simulink library "tether001_cl"  (R2020a)
settings: Solver=VariableStepAuto  StartTime=0.0  StopTime=10.0  RelTol=1e-3
undefined symbols (not defined in the file or in its folder): env, initNodePos, minLinkDeviation, minLinkLength, minSoftLength, numNodes, thr
libraries: powerlib_meascontrol x1, nodePosToLinkPos_ul x1
settings Model: Creator=mr-jo  LastModifiedBy=John Jr

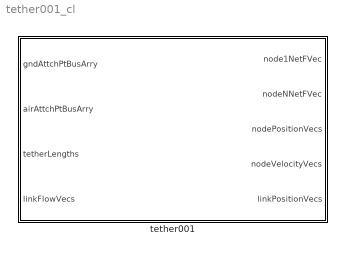
== system tether001_cl ==
  tether001 : Subsystem  mask{thr=thr.tether1, fluidDensity=env.water.density.Value, gravity=env.gravAccel.Value}
      mask prompts: thr "Tether001 Object"; fluidDensity "Fluid Density"; gravity "Gravitational Aceleration"

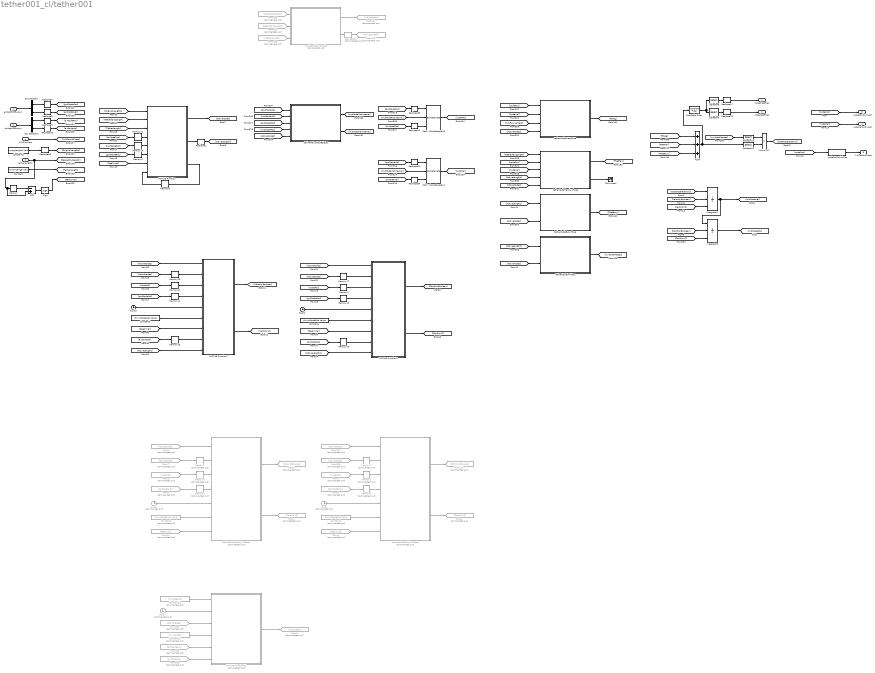
== system tether001_cl/tether001 ==
  gndAttchPtBusArry : Inport  OutDataTypeStr=Bus: thrAttachPtKinematicsBus
  airAttchPtBusArry : Inport  Port=2  OutDataTypeStr=Bus: thrAttachPtKinematicsBus
  tetherLengths : Inport  Port=3
  linkFlowVecs : Inport  Port=4
  Add : Sum  Inputs=-+
  Add4 : Sum  Inputs=3
  Bus Selector : BusSelector  OutputSignals=posVec,velVec
  Bus Selector1 : BusSelector  OutputSignals=posVec,velVec
  Clock : Clock  Commented=on
  Clock1 : Clock  Commented=on
  Clock2 : Clock
  Clock3 : Clock
  Clock7 : Clock  Commented=on
  Constant : Constant  Value=thr.maxLength.Value
  Constant1 : Constant  Commented=on  Value=thr.initNodePos.Value
  Constant15 : Constant  Commented=on  Value=[initNodePos]
  Constant19 : Constant  Commented=on  Value=[numNodes]
  Constant2 : Constant  Commented=on  Value=thr.initNodeVel.Value
  Constant3 : Constant  Value=thr.orgLengths.Value
  Constant4 : Constant  Value=thr.initNodePos.Value
  Constant5 : Constant  Value=thr.initNodeVel.Value
  First-Order Filter : powerlib_meascontrol/Filters/First-Order Filter  FilterType=Lowpass  Tc=10e-2  Ts=0  Initialize=on  Vac_Init=[0, 0, 60]  Vdc_Init=0  PlotResponse=off  FreqRange="[0,  200,  1]"
  From1 : From  Commented=on  GotoTag=nodePos
  From10 : From  Commented=on  GotoTag=ReelInVel
  From161 : From  Commented=on  GotoTag=gndNodePos
  From162 : From  Commented=on  GotoTag=airNodePos
  From2 : From  Commented=on  GotoTag=gndNodePos
  From{4,7,267..268,361} (5 alike) : From  Commented=on  GotoTag=ActiveNodes
  From310 : From  Commented=on  GotoTag=OriginalLengths
  From311 : From  Commented=on  GotoTag=ReeledOutLength
  From320 : From  Commented=on  GotoTag=TetherLength
  From5 : From  Commented=on  GotoTag=ReelInVel
  From8 : From  Commented=on  GotoTag=nodeVel
  From9 : From  Commented=on  GotoTag=gndNodeVel
  Goto110 : Goto  Commented=on  GotoTag=PositionBoolean
  Goto152 : Goto  Commented=on  GotoTag=ActiveLengths
  Goto161 : Goto  Commented=on  GotoTag=ActiveNodes
  Goto2 : Goto  Commented=on  GotoTag=PositionIC
  Goto3 : Goto  Commented=on  GotoTag=VelocityBoolean
  Goto4 : Goto  Commented=on  GotoTag=VelocityIC
  Goto5 : Goto  Commented=on  GotoTag=PosIC_Start
  Integrator1 : Integrator  ExternalReset=rising  InitialConditionSource=external
  Integrator8 : Integrator  ExternalReset=rising  InitialConditionSource=external
  MATLAB Function : MATLAB Function  TreatAsAtomicUnit=on  mask{minLinkLength=minLinkLength, minLinkDeviation=minLinkDeviation}
      mask prompts: minLinkLength "Minimum Link Length"; minLinkDeviation "Minimum Devation to Remove Node"
  MATLAB Function1 : MATLAB Function  TreatAsAtomicUnit=on
  MATLAB Function2 : MATLAB Function  TreatAsAtomicUnit=on
  MATLAB Function61 : MATLAB Function  Commented=on  TreatAsAtomicUnit=on
  Matrix Concatenate14 : Concatenate  NumInputs=3  Mode=Multidimensional array  ConcatenateDimension=2
  Matrix Concatenate15 : Concatenate  NumInputs=3  Mode=Multidimensional array  ConcatenateDimension=2
  Memory{,6,8..18} (13 alike) : Memory
  Memory{1..5,7} (6 alike) : Memory  Commented=on
  Multiply11 : Product
  Reshape1 : Reshape  OutputDimensionality=Row vector (2-D)
  Reshape{7..10,17..18,33..34,41..42} (10 alike) : Reshape  OutputDimensionality=Column vector (2-D)
  Reshape36 : Reshape  OutputDimensionality=Row vector (2-D)
  Reshape39 : Reshape  Commented=on  OutputDimensionality=Row vector (2-D)
  Selector18 : Selector  NumberOfDimensions=2  InputPortWidth=3  IndexOptions=Select all,Index vector (dialog)  Indices=[1 3],2:thr.numNodes.Value-1  OutputSizes=1,1
  Selector19 : Selector  NumberOfDimensions=2  InputPortWidth=3  IndexOptions=Select all,Index vector (dialog)  Indices=[1 3],2:thr.numNodes.Value-1  OutputSizes=1,1
  Selector8 : Selector  NumberOfDimensions=2  InputPortWidth=3  IndexOptions=Select all,Index vector (dialog)  Indices=[1 3],1  OutputSizes=1,1
  Selector9 : Selector  NumberOfDimensions=2  InputPortWidth=3  IndexOptions=Select all,Starting index (dialog)  Indices=[1 3],thr.numNodes.Value  OutputSizes=1,1
  Sign : Signum
  Terminator : Terminator
  defineActiveNodeStates : MATLAB Function  TreatAsAtomicUnit=on
  nodePosToLinkPos : nodePosToLinkPos_ul/nodePosToLinkPos  SystemSampleTime=-1  Latency=0  AutoFrameSizeCalculation=off
  numberOfActiveNodes : MATLAB Function  Commented=on  TreatAsAtomicUnit=on
  tetherNodeBuoyForce : MATLAB Function  TreatAsAtomicUnit=on  mask{fluidDensity=fluidDensity, numNodes=thr.numNodes.Value, thrDiam=thr.diameter.Value, tetherDensity=thr.density.Value, gravity=gravity}
      mask prompts: fluidDensity "Fluid Density"; numNodes "Number of Nodes"; thrDiam "Tether Diameter"; tetherDensity "Tether Density"; gravity "Gravitational Acceleration"
  tetherNodeDragForce : MATLAB Function  TreatAsAtomicUnit=on  mask{flowDensity=fluidDensity, numNodes=thr.numNodes.Value, dragCoeff=thr.dragCoeff.Value, thrDiam=thr.diameter.Value}
      mask prompts: flowDensity "Fluid Density"; numNodes "Number of nodes"; dragCoeff "Drag Coefficient of Tether"; thrDiam "Tether Diameter"
  tetherNodeInvMass : MATLAB Function  TreatAsAtomicUnit=on  mask{numNodes=thr.numNodes.Value, thrDiam=thr.diameter.Value, tetherDensity=thr.density.Value}
      mask prompts: numNodes "Number of nodes"; thrDiam "Tether Diameter"; tetherDensity "Tether Density"
  tetherNodePositionICReset : MATLAB Function  Commented=on  TreatAsAtomicUnit=on
  tetherNodeTensionForce : MATLAB Function  TreatAsAtomicUnit=on  mask{numNodes=thr.numNodes.Value, thrDiam=thr.diameter.Value, youngsMod=thr.youngsMod.Value, dampingRatio=thr.dampingRatio.Value, mass=thr.vehicleMass.Value, minSoftLength=minSoftLength}
      mask prompts: numNodes "Number of Nodes"; thrDiam "Tether Diameter"; youngsMod "Youngs Modulus of Tether"; dampingRatio "Total Tether Damping Ratio"; mass "Vehicle Mass for Damping"; minSoftLength "Min Link Length for Spring Softening"
  tetherNodeVelocityICReset : MATLAB Function  Commented=on  TreatAsAtomicUnit=on
  node1NetFVec : Outport  VectorParamsAs1DForOutWhenUnconnected=off
  nodeNNetFVec : Outport  Port=2  VectorParamsAs1DForOutWhenUnconnected=off
  nodePositionVecs : Outport  Port=3  VectorParamsAs1DForOutWhenUnconnected=off
  nodeVelocityVecs : Outport  Port=4  VectorParamsAs1DForOutWhenUnconnected=off
  linkPositionVecs : Outport  Port=5  VectorParamsAs1DForOutWhenUnconnected=off
  wires:
  [nodePos] -> nodePosToLinkPos/1
  nodePosToLinkPos/1 -> linkPositionVecs/1  "linkPositions"
  [nodeVel] -> nodeVelocityVecs/1
  [nodePos] -> nodePositionVecs/1
  Constant3/1 -> Reshape36/1
  Sign/1 -> [ReelInVel]
  Add/1 -> Sign/1
  Memory/1 -> Add/1
  Bus Selector/1 -> Reshape7/1  "<posVec>"
  Reshape8/1 -> [gndNodeVel]
  Bus Selector1/1 -> Reshape9/1  "<posVec>"
  Bus Selector/2 -> Reshape8/1  "<velVec>"
  airAttchPtBusArry/1 -> Bus Selector1/1
  Reshape9/1 -> [airNodePos]
  Reshape10/1 -> [airNodeVel]
  Reshape7/1 -> [gndNodePos]
  gndAttchPtBusArry/1 -> Bus Selector/1
  Bus Selector1/2 -> Reshape10/1  "<velVec>"
  Constant1/1 -> tetherNodePositionICReset/6(GivenIC)
  MATLAB Function61/1(PosIC_Start) -> Goto5/1
  Constant15/1 -> MATLAB Function61/1(initNodePos)
  From161/1 -> MATLAB Function61/5(gndNodePos)
  Clock7/1 -> MATLAB Function61/2(time)
  From162/1 -> MATLAB Function61/6(airNodePos)
  Constant19/1 -> MATLAB Function61/4(OriginalNodes)
  From361/1 -> MATLAB Function61/3(ActiveNodes)
  Memory1/1 -> tetherNodePositionICReset/3(nodePositions)
  From1/1 -> Memory1/1
  [ActiveNodes] -> tetherNodeInvMass/2(ActiveNodes)
  [ActiveLengths] -> tetherNodeBuoyForce/1(ActiveLengths)
  [VelocityBoolean] -> Integrator1/2
  [VelocityIC] -> Integrator1/3
  tetherNodeVelocityICReset/2(VelocityIC) -> Goto4/1
  tetherNodeVelocityICReset/1(Bool) -> Goto3/1
  From10/1 -> tetherNodeVelocityICReset/7(ReelInVel)
  Constant2/1 -> tetherNodeVelocityICReset/6(GivenIC)
  Clock1/1 -> tetherNodeVelocityICReset/5(time)
  Memory5/1 -> tetherNodeVelocityICReset/4(gndNodeVel)
  From9/1 -> Memory5/1
  Memory4/1 -> tetherNodeVelocityICReset/3(nodeVelocities)
  From8/1 -> Memory4/1
  Memory2/1 -> tetherNodeVelocityICReset/2(PrevStepNumNodes)
  From7/1 -> Memory2/1
  From4/1 -> tetherNodeVelocityICReset/1(CurStepNumNodes)
  [PositionBoolean] -> Integrator8/2
  Selector9/1 -> Reshape18/1
  Selector8/1 -> Reshape17/1
  From5/1 -> tetherNodePositionICReset/7(ReelInVel)
  Memory3/1 -> tetherNodePositionICReset/4(gndNodePos)
  [PositionIC] -> Integrator8/3
  Clock/1 -> tetherNodePositionICReset/5(time)
  tetherNodePositionICReset/2(PositionIC) -> Goto2/1
  From2/1 -> Memory3/1
  [NodeAccelerations] -> Integrator1/1
  [FNetBuoy] -> Add4/3  "FbuoyT"
  Multiply11/1 -> [NodeAccelerations]
  [FDrag] -> Add4/1  "FdragT"
  Selector19/1 -> Multiply11/1
  [invNodeMasses] -> Selector19/1
  Memory7/1 -> tetherNodePositionICReset/2(PrevStepNumNodes)
  From268/1 -> Memory7/1
  tetherNodePositionICReset/1(Bool) -> Goto110/1
  From267/1 -> tetherNodePositionICReset/1(CurStepNumNodes)
  defineActiveNodeStates/1(midNodePosInternal) -> [midNodePosInternal]
  Constant/1 -> [TetherLength]
  linkFlowVecs/1 -> [linkFlowVelVecs]
  Reshape36/1 -> [OriginalLengths]
  tetherLengths/1 -> [ReeledOutLength], Memory/1, Add/2
  From310/1 -> numberOfActiveNodes/1(OriginalLengths)
  [linkFlowVelVecs] -> tetherNodeDragForce/3(flowVel)
  [midNodeVel] -> defineActiveNodeStates/2(midNodeVel)
  [nodePos] -> tetherNodeTensionForce/2(nodePos)
  defineActiveNodeStates/2(midNodeVelInternal) -> [midNodeVelInternal]
  [ReeledOutLength] -> tetherNodeTensionForce/1(ReeledOutLength)
  [ActiveNodes] -> tetherNodeDragForce/4(NumberNodesActive)
  From320/1 -> numberOfActiveNodes/3(TetherLength)
  [nodeVel] -> tetherNodeDragForce/2(nodeVelocities)
  Reshape34/1 -> Matrix Concatenate14/3
  [gndNodePos] -> defineActiveNodeStates/3(gndNodePos)
  [midNodeVelInternal] -> Matrix Concatenate14/2
  [ActiveNodes] -> defineActiveNodeStates/5(ActiveNodes)
  [midNodePos] -> defineActiveNodeStates/4(midNodePos)
  numberOfActiveNodes/1(ActiveNodes) -> Goto161/1
  [gndNodeVel] -> defineActiveNodeStates/1(gndNodeVel)
  [ActiveLengths] -> tetherNodeTensionForce/4(ActiveLengths)
  Matrix Concatenate15/1 -> [nodePos]
  tetherNodeTensionForce/1(nodeForceVecs) -> [FNetTen]
  Matrix Concatenate14/1 -> [nodeVel]
  [nodeVel] -> tetherNodeTensionForce/3(nodeVel)
  [airNodeVel] -> Reshape34/1
  Reshape33/1 -> Matrix Concatenate15/1
  Reshape41/1 -> Matrix Concatenate15/3
  Reshape39/1 -> Goto152/1
  [ActiveNodes] -> tetherNodeBuoyForce/2(NumberNodesActive)
  Reshape42/1 -> Matrix Concatenate14/1
  From311/1 -> numberOfActiveNodes/2(ReeledOutLength)
  tetherNodeBuoyForce/1(nodeForceVecs) -> [FNetBuoy]
  [ActiveLengths] -> tetherNodeInvMass/1(Activelength)
  [nodePos] -> tetherNodeDragForce/1(nodePositions)
  [midNodePosInternal] -> Matrix Concatenate15/2
  [airNodePos] -> Reshape41/1
  numberOfActiveNodes/2(ActiveLengths) -> Reshape39/1
  [gndNodePos] -> Reshape33/1
  tetherNodeInvMass/1(invNodeMasses) -> [invNodeMasses]
  [ActiveNodes] -> tetherNodeTensionForce/5(NumberNodesActive)
  [gndNodeVel] -> Reshape42/1
  tetherNodeDragForce/1(nodeForceVecs) -> [FDrag]
  [gndNodePos] -> Memory8/1
  Memory6/1 -> MATLAB Function/8(FirstLinkPrev)
  Memory11/1 -> MATLAB Function/4(airNodePos)
  Memory10/1 -> MATLAB Function/5(midNodePos)
  Memory8/1 -> MATLAB Function/6(gndNodePos)
  MATLAB Function/3(FirstLink) -> Memory6/1
  [TetherLength] -> MATLAB Function/3(TetherLength)
  [airNodePos] -> Memory11/1
  [OriginalLengths] -> MATLAB Function/1(OriginalLengths)
  [ReelInVel] -> MATLAB Function/7(ReelInVel)
  [ReeledOutLength] -> MATLAB Function/2(ReeledOutLength)
  MATLAB Function/2(ActiveLengths) -> Reshape1/1
  MATLAB Function/1(ActiveNodes) -> [ActiveNodes]
  [midNodePos] -> Memory10/1
  Reshape1/1 -> [ActiveLengths]
  [ActiveLengths] -> MATLAB Function2/9(ActiveLengths)
  [ReelInVel] -> MATLAB Function1/7(ReelInVel)
  Memory12/1 -> MATLAB Function2/3(nodeVelocities)
  MATLAB Function2/1(Bool) -> [VelocityBoolean]
  Memory9/1 -> MATLAB Function1/3(nodePositions)
  [airNodePos] -> Memory16/1
  Memory15/1 -> MATLAB Function2/8(airNodePos)
  [ActiveNodes] -> MATLAB Function1/1(CurStepNumNodes)
  [ActiveLengths] -> MATLAB Function1/9(ActiveLengths)
  [nodePos] -> Memory9/1
  Memory14/1 -> MATLAB Function2/4(gndNodeVel)
  Constant5/1 -> MATLAB Function2/6(GivenIC)
  Memory18/1 -> MATLAB Function2/2(PrevStepNumNodes)
  [gndNodeVel] -> Memory14/1
  [ReelInVel] -> MATLAB Function2/7(ReelInVel)
  [nodeVel] -> Memory12/1
  Memory17/1 -> MATLAB Function1/2(PrevStepNumNodes)
  [gndNodePos] -> Memory13/1
  Clock3/1 -> MATLAB Function2/5(time)
  MATLAB Function1/2(PositionIC) -> [PositionIC]
  [airNodeVel] -> Memory15/1
  Memory13/1 -> MATLAB Function1/4(gndNodePos)
  MATLAB Function2/2(VelocityIC) -> [VelocityIC]
  Clock2/1 -> MATLAB Function1/5(time)
  Memory16/1 -> MATLAB Function1/8(airNodePos)
  [ActiveNodes] -> MATLAB Function2/1(CurStepNumNodes)
  MATLAB Function1/1(Bool) -> [PositionBoolean]
  Constant4/1 -> MATLAB Function1/6(GivenIC)
  [ActiveNodes] -> Memory17/1
  [ActiveNodes] -> Memory18/1
  Reshape17/1 -> node1NetFVec/1  "node1NetFVec"
  Reshape18/1 -> nodeNNetFVec/1  "nodeNNetFVec"
  tetherNodeTensionForce/2(Scope) -> Terminator/1  "Scope"
  [FNetTen] -> Add4/2  "FtenT"
  First-Order Filter/1 -> Selector8/1, Selector9/1
  Add4/1 -> Selector18/1, First-Order Filter/1
  Selector18/1 -> Multiply11/2
  Integrator1/1 -> Integrator8/1, [midNodeVel]
  Integrator8/1 -> [midNodePos]

== matlab function tether001_cl/tether001/defineActiveNodeStates ==
  data: gndNodeVel input size=[3,1]; midNodeVel input size=[3,thr.numNodes.Value-2]; gndNodePos input size=[3,1]; midNodePosInternal output size=[3,thr.numNodes.Value-2]; midNodePos input size=[3,thr.numNodes.Value-2]; ActiveNodes input size=1; midNodeVelInternal output size=[3,thr.numNodes.Value-2]
function [midNodePosInternal,  midNodeVelInternal] = fcn(gndNodeVel,midNodeVel,gndNodePos, midNodePos, ActiveNodes)

No = size(midNodePos,2)+2;
Na = ActiveNodes;

% Reeled In Nodes are ground
midNodePosInternal = [gndNodePos(1)*ones(1,No-2);...
                      gndNodePos(2)*ones(1,No-2);...
                      gndNodePos(3)*ones(1,No-2)];
                  
midNodeVelInternal = [gndNodeVel(1)*ones(1,No-2);...
                      gndNodeVel(2)*ones(1,No-2);...
                      gndNodeVel(3)*ones(1,No-2)];              
                  
% Given for unalternd nodes
midNodePosInternal(:,((No-Na)+1):end) = midNodePos(:,((No-Na)+1):end);
midNodeVelInternal(:,((No-Na)+1):end) = midNodeVel(:,((No-Na)+1):end);

== matlab function tether001_cl/tether001/tetherNodeInvMass ==
  data: invNodeMasses output size=[3,thr.numNodes.Value]; Activelength input; ActiveNodes input; numNodes parameter; thrDiam parameter; tetherDensity parameter
function invNodeMasses  = fcn(Activelength,ActiveNodes, numNodes, thrDiam, tetherDensity)
    invNodeMasses  = tetherNodeInvMass(Activelength,ActiveNodes, numNodes, thrDiam, tetherDensity);
end

== matlab function tether001_cl/tether001/tetherNodeDragForce ==
  data: nodePositions input size=[3,thr.numNodes.Value]; nodeVelocities input size=[3,thr.numNodes.Value]; flowVel input size=[3,thr.numNodes.Value-1]; NumberNodesActive input size=1; nodeForceVecs output size=[3,thr.numNodes.Value]; numNodes parameter size=1; dragCoeff parameter; thrDiam parameter; flowDensity parameter
function nodeForceVecs = fcn(nodePositions,nodeVelocities, flowVel, NumberNodesActive, numNodes, dragCoeff, thrDiam, flowDensity)
    nodeForceVecs = tetherNodeDragForce(nodePositions,nodeVelocities, flowVel, NumberNodesActive, numNodes, dragCoeff, thrDiam, flowDensity);
end

== matlab function tether001_cl/tether001/tetherNodeBuoyForce ==
  data: ActiveLengths input; NumberNodesActive input; nodeForceVecs output size=[3,thr.numNodes.Value]; numNodes parameter; thrDiam parameter; tetherDensity parameter; gravity parameter; fluidDensity parameter
function nodeForceVecs = fcn(ActiveLengths, NumberNodesActive, numNodes, thrDiam, tetherDensity, gravity, fluidDensity)
    nodeForceVecs = tetherNodeBuoyForce(ActiveLengths, NumberNodesActive, numNodes, thrDiam, tetherDensity, gravity, fluidDensity);
end

== matlab function tether001_cl/tether001/tetherNodeVelocityICReset ==
  data: CurStepNumNodes input; Bool output; PrevStepNumNodes input; nodeVelocities input; gndNodeVel input; time input; GivenIC input; ReelInVel input; VelocityIC output
function [Bool,VelocityIC]  = fcn(CurStepNumNodes, PrevStepNumNodes, nodeVelocities, gndNodeVel, time, GivenIC, ReelInVel)
    [Bool,VelocityIC]  = tetherNodeVelocityICReset(CurStepNumNodes, PrevStepNumNodes, nodeVelocities, gndNodeVel, time, GivenIC, ReelInVel);
end

== matlab function tether001_cl/tether001/MATLAB Function61 ==
  data: initNodePos input size=[3,numNodes-2]; time input size=1; ActiveNodes input size=1; OriginalNodes input size=1; gndNodePos input size=[3,1]; airNodePos input size=[3,1]; PosIC_Start output
function PosIC_Start = fcn(initNodePos,time, ActiveNodes, OriginalNodes,gndNodePos,airNodePos)

if time==0
    Na = ActiveNodes;
    No = 11;%OriginalNodes;
    
    TetherVec = [linspace(gndNodePos(1),airNodePos(1),Na);...
                 linspace(gndNodePos(2),airNodePos(2),Na);...
                 linspace(gndNodePos(3),airNodePos(3),Na)];
    PosIC_Start = [gndNodePos(1)*ones(1,No-2);...
             gndNodePos(2)*ones(1,No-2);...
             gndNodePos(3)*ones(1,No-2)];

    % initNodePos   
    PosIC_Start(1,((No-Na)+1):end) = linspace(TetherVec(1,2),TetherVec(1,end-1),Na-2);
    PosIC_Start(2,((No-Na)+1):end) = linspace(TetherVec(2,2),TetherVec(2,end-1),Na-2);
    PosIC_Start(3,((No-Na)+1):end) = linspace(TetherVec(3,2),TetherVec(3,end-1),Na-2);
else
    PosIC_Start = zeros(3,size(initNodePos,2));
end

== matlab function tether001_cl/tether001/tetherNodePositionICReset ==
  data: CurStepNumNodes input; Bool output; PrevStepNumNodes input; nodePositions input; gndNodePos input; PositionIC output; time input; GivenIC input; ReelInVel input
function [Bool,PositionIC]  = fcn(CurStepNumNodes, PrevStepNumNodes, nodePositions, gndNodePos, time, GivenIC, ReelInVel)
    [Bool,PositionIC]  = tetherNodePositionICReset(CurStepNumNodes, PrevStepNumNodes, nodePositions, gndNodePos, time, GivenIC, ReelInVel);
end

== matlab function tether001_cl/tether001/MATLAB Function1 ==
  data: CurStepNumNodes input; Bool output; PrevStepNumNodes input; nodePositions input; gndNodePos input; time input; GivenIC input; ReelInVel input; airNodePos input; ActiveLengths input; PositionIC output
function [Bool,PositionIC]  = fcn(CurStepNumNodes, PrevStepNumNodes, nodePositions, gndNodePos, time, GivenIC, ReelInVel, airNodePos, ActiveLengths)

if ReelInVel<=0
    if time==0
        PositionIC = GivenIC;
        Bool = 1;
    else
        Na = CurStepNumNodes;
        No = size(nodePositions,2);

        if PrevStepNumNodes==0
            Nc = CurStepNumNodes;
            Np = Nc;
        else
            Np = PrevStepNumNodes;
            Nc = CurStepNumNodes;
        end

        PositionIC = [gndNodePos(1)*ones(1,No-2);...
                      gndNodePos(2)*ones(1,No-2);...
                      gndNodePos(3)*ones(1,No-2)];
        if Nc == Np
            Bool = -1;
        else
            Bool = 1;
            PositionIC(:,(No-Na+1):end) = nodePositions(:,(No-Na+2):end-1);
        end
    end         
else
    if time==0
        PositionIC = GivenIC;
        Bool = 1;
    else
        Na = CurStepNumNodes;
        No = size(nodePositions,2);

        if PrevStepNumNodes==0
            Nc = CurStepNumNodes;
            Np = Nc;
        else
            Np = PrevStepNumNodes;
            Nc = CurStepNumNodes;
        end

        PositionIC = [gndNodePos(1)*ones(1,No-2);...
                      gndNodePos(2)*ones(1,No-2);...
                      gndNodePos(3)*ones(1,No-2)];
        if Nc == Np
            Bool = -1;
        else
            Bool = 1;
            linkVecs  = diff(nodePositions,1,2);
            linkVecsUnit = linkVecs./repmat(sqrt(sum((linkVecs.^2),1)),[3 1]);
            linkVecsUnit(isnan(linkVecsUnit))=0;
            PositionIC(:,(No-Na+2):end) = nodePositions(:,(No-Na+3):end-1);
            PositionIC(:,(No-Na+1)) = linkVecsUnit(:,(No-Na+1)).*ActiveLengths(:,No-Na+1);
        end
    end
end

== matlab function tether001_cl/tether001/MATLAB Function ==
  data: OriginalLengths input; ActiveNodes output; ReeledOutLength input; TetherLength input; airNodePos input; midNodePos input; gndNodePos input; ReelInVel input; FirstLinkPrev input; ActiveLengths output; FirstLink output; minLinkLength parameter; minLinkDeviation parameter
function [ActiveNodes, ActiveLengths,FirstLink] = fcn(OriginalLengths, ReeledOutLength, TetherLength,airNodePos, midNodePos, gndNodePos,ReelInVel,FirstLinkPrev,minLinkLength, minLinkDeviation)
    [ActiveNodes, ActiveLengths,FirstLink] = numberOfActiveNodes(OriginalLengths, ReeledOutLength, TetherLength,airNodePos, midNodePos, gndNodePos,ReelInVel,FirstLinkPrev,minLinkLength,minLinkDeviation);
end

== matlab function tether001_cl/tether001/MATLAB Function2 ==
  data: CurStepNumNodes input; Bool output; PrevStepNumNodes input; nodeVelocities input; gndNodeVel input; time input; GivenIC input; ReelInVel input; airNodePos input; ActiveLengths input; VelocityIC output
function [Bool,VelocityIC]  = fcn(CurStepNumNodes, PrevStepNumNodes, nodeVelocities, gndNodeVel, time, GivenIC, ReelInVel, airNodePos, ActiveLengths)

if ReelInVel<=0
    if time==0
        VelocityIC = GivenIC;
        Bool = 1;
    else
        Na = CurStepNumNodes;
        No = size(nodeVelocities,2);

        if PrevStepNumNodes==0
            Nc = CurStepNumNodes;
            Np = Nc;
        else
            Np = PrevStepNumNodes;
            Nc = CurStepNumNodes;
        end

        VelocityIC = [gndNodeVel(1)*ones(1,No-2);...
                      gndNodeVel(2)*ones(1,No-2);...
                      gndNodeVel(3)*ones(1,No-2)];
        if Nc == Np
            Bool = -1;
        else
            Bool = 1;
            VelocityIC(:,(No-Na+1):end) = nodeVelocities(:,(No-Na+2):end-1);
        end
    end         
else
    if time==0
        VelocityIC = GivenIC;
        Bool = 1;
    else
        Na = CurStepNumNodes;
        No = size(nodeVelocities,2);

        if PrevStepNumNodes==0
            Nc = CurStepNumNodes;
            Np = Nc;
        else
            Np = PrevStepNumNodes;
            Nc = CurStepNumNodes;
        end

        VelocityIC = [gndNodeVel(1)*ones(1,No-2);...
                      gndNodeVel(2)*ones(1,No-2);...
                      gndNodeVel(3)*ones(1,No-2)];
        if Nc == Np
            Bool = -1;
        else
            Bool = 1;
            linkVecs  = diff(nodeVelocities,1,2);
            linkVecsUnit = linkVecs./repmat(sqrt(sum((linkVecs.^2),1)),[3 1]);
            linkVecsUnit(isnan(linkVecsUnit))=0;
            VelocityIC(:,(No-Na+2):end) = nodeVelocities(:,(No-Na+3):end-1);
            VelocityIC(:,(No-Na+1)) = linkVecsUnit(:,(No-Na+1)).*ActiveLengths(:,No-Na+1);
        end
    end
end

== matlab function tether001_cl/tether001/numberOfActiveNodes ==
  data: OriginalLengths input; ActiveNodes output; ReeledOutLength input; ActiveLengths output; TetherLength input
function [ActiveNodes, ActiveLengths] = fcn(OriginalLengths, ReeledOutLength, TetherLength)
    [ActiveNodes, ActiveLengths] = numberOfActiveNodes(OriginalLengths, ReeledOutLength, TetherLength);
end

== matlab function tether001_cl/tether001/tetherNodeTensionForce ==
  data: ReeledOutLength input; nodePos input; nodeForceVecs output size=[3,thr.numNodes.Value]; nodeVel input; ActiveLengths input; NumberNodesActive input; numNodes parameter; thrDiam parameter; youngsMod parameter; dampingRatio parameter; mass parameter; minSoftLength parameter; Scope output size=[1,8]
function [nodeForceVecs,Scope]   = fcn(ReeledOutLength, nodePos, nodeVel, ActiveLengths, NumberNodesActive, numNodes, thrDiam, youngsMod, dampingRatio, mass, minSoftLength)
    [nodeForceVecs,Scope]  = tetherNodeTensionForce(ReeledOutLength, nodePos, nodeVel, ActiveLengths, NumberNodesActive, numNodes, thrDiam, youngsMod, dampingRatio, mass, minSoftLength);
end
